simulink model "Symmetry_COPY"  (Simulink 8.1)
settings: Solver=ode23t  StartTime=0.0  StopTime=tfin  RelTol=1e-4
values from neighbouring files (symbols this model uses):
  amp_feedback_saturation = 400    [Symmetry_ini_COPY.m]
  Butterworth_filter_order = 8    [Sketch_controller_model_ini.m]    (also in Symmetry_ini.m; Symmetry_ini_COPY.m)
  C_Network = [0, 0, 0]    [Symmetry_ini.m]    (also in Symmetry_ini_COPY.m)
  Capacitive_Load_R_RC = [30e-3,  60e-3,  40e-3;                                1e-3, 5e-3, 3e-3]    [Symmetry_ini.m]    (also in Symmetry_ini_COPY.m = [60e-3,  120e-3,  80e-3;                                1e-3)
  Capacitive_Load_R_Switching_Sequence = Capacitive_Load_R_Switching_Sequence_'    [Symmetry_ini.m]    (also in Symmetry_ini_COPY.m = ones(3,tfin/Capacitive_Load_R_Switching_Speed(1))')
  Capacitive_Load_R_Switching_Speed = [0.01,0.01,0.01]    [Symmetry_ini.m]    (also in Symmetry_ini_COPY.m)
  Capacitive_Load_S_RC = [30e-3,  60e-3,  40e-3;                                1e-3, 5e-3, 3e-3]    [Symmetry_ini.m]    (also in Symmetry_ini_COPY.m = [60e-3,  120e-3,  80e-3;                                1e-3)
  Capacitive_Load_S_Switching_Sequence = Capacitive_Load_S_Switching_Sequence_'    [Symmetry_ini.m]    (also in Symmetry_ini_COPY.m = ones(3,tfin/Capacitive_Load_R_Switching_Speed(1))')
  Capacitive_Load_S_Switching_Speed = [0.01,0.01,0.01]    [Symmetry_ini.m]    (also in Symmetry_ini_COPY.m)
  Capacitive_Load_T_RC = [30e-3,  60e-3,  40e-3;                                1e-3, 5e-3, 3e-3]    [Symmetry_ini.m]    (also in Symmetry_ini_COPY.m = [60e-3,  120e-3,  80e-3;                                1e-3)
  Capacitive_Load_T_Switching_Sequence = Capacitive_Load_T_Switching_Sequence_'    [Symmetry_ini.m]    (also in Symmetry_ini_COPY.m = ones(3,tfin/Capacitive_Load_R_Switching_Speed(1))')
  Capacitive_Load_T_Switching_Speed = [0.01,0.01,0.01]    [Symmetry_ini.m]    (also in Symmetry_ini_COPY.m)
  i = str2num(answer{1})/sample    [Test_intersect.m]
  initial_value = [1,1,1,                  0,-2/3*pi,-4/3*pi]    [Symmetry_ini_COPY.m]
  L_Network = [3.185e-3, 3.185e-3, 3.185e-3, 3.185e-3]    [Symmetry_ini.m]    (also in Symmetry_ini_COPY.m)
  L_Source = [3.185e-3, 3.185e-3, 3.185e-3]    [Sketch_controller_model_ini.m]    (also in Symmetry_ini.m; Symmetry_ini_COPY.m)
  Load_R = [50,50,50]    [Symmetry_ini.m]    (also in Symmetry_ini_COPY.m)
  Load_RL = [35.35,   35.35,   35.35;                  0.1125,  0.1125,  0.1125]    [Symmetry_ini.m]    (also in Symmetry_ini_COPY.m)
  Load_Wire_Resistance = [0.1,0.2]    [Symmetry_ini.m]    (also in Symmetry_ini_COPY.m)
  P_gain = 0.01    [Symmetry_ini_COPY.m]
  phase_feedback_saturation = pi    (= 3.14159265359)    [Symmetry_ini_COPY.m]
  Phase_Source = [0,2/3*pi,4/3*pi]    [Sketch_controller_model_ini.m]    (also in Symmetry_REAL_TIME_ini.m = [0,-2/3*pi,-4/3*pi]; Symmetry_ini.m; Symmetry_ini_COPY.m = [0,-2/3*pi,-4/3*pi])
  R_Network = [0.4, 0.4, 0.4, 0.4]    [Symmetry_ini.m]    (also in Symmetry_ini_COPY.m)
  R_Source = [0.4, 0.4, 0.4]    [Sketch_controller_model_ini.m]    (also in Symmetry_ini.m; Symmetry_ini_COPY.m)
  sample = 10e-5    (= 0.0001)    [Inverter_ini.m]    (also in Sketch_controller_model_ini.m; Symmetry_REAL_TIME_ini.m; Symmetry_ini.m; Symmetry_ini_COPY.m)
  Source_Frequency = [50,50,50]    [Sketch_controller_model_ini.m]    (also in Symmetry_ini.m; Symmetry_ini_COPY.m)
  Start_Control = 0.1    [Symmetry_ini_COPY.m]
  step_size = [5,5,5,                  0.32,0.32,0.32]    [Symmetry_ini_COPY.m]
  Switch_Load_R = [1,1,1]    [Symmetry_ini.m]    (also in Symmetry_ini_COPY.m = [1,0,0])
  Switch_Load_RC = [1,1,1]    [Symmetry_ini.m]    (also in Symmetry_ini_COPY.m = [0,0,1])
  Switch_Load_RL = [1,1,1]    [Symmetry_ini.m]    (also in Symmetry_ini_COPY.m = [0,1,0])
  test_step = [1,1,1,                  0.08,0.08,0.08]    [Symmetry_ini_COPY.m]
  Urms_Source = [230,230,230]    [Sketch_controller_model_ini.m]    (also in Symmetry_REAL_TIME_ini.m; Symmetry_ini.m; Symmetry_ini_COPY.m)
libraries: powerlib x87, simulink x27, powerlib_extras x12, dspsigops x10, commsequence2 x6, dspxfrm3 x3, dsparch4 x3
(part 1 of 2)
settings Model: Creator=gorbep  LastModifiedBy=Neukirchner László
settings SolverCC: ZeroCrossControl=EnableAll  ZeroCrossAlgorithm=Adaptive  SolverResetMethod=Robust
settings DataIOCC: SignalLoggingSaveFormat=Dataset
settings OptimizationCC: ExpressionDepthLimit=128
settings DebuggingCC: UnderspecifiedInitializationDetection=Simplified  FcnCallInpInsideContextMsg=EnableAllAsError  StateNameClashWarn=none
settings GRTTargetCC: CodeReplacementLibrary=None  CombineOutputUpdateFcns=on  CPPClassGenCompliant=on  GRTInterface=off

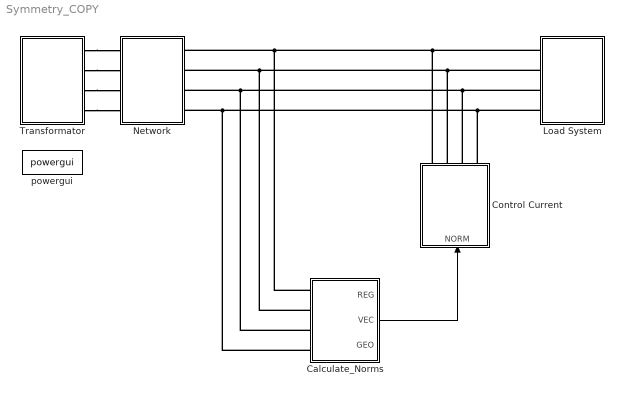
== system Symmetry_COPY ==
  Calculate_Norms : Subsystem
  Control Current : Subsystem
  Load System : Subsystem
  Network : Subsystem
  Transformator : Subsystem
  powergui : powerlib/powergui  SimulationMode=Continuous  SolverType=Tustin  SampleTime=50e-6  frequency=60  SPID=off  DisableSnubberDevices=off  DisableRonSwitches=off  DisableVfSwitches=off  SwTol=0  Interpol=off  DisplayEquations=off  frequencyindice=0  Pbase=100e6  ErrMax=1e-4  Iterations=50  UnitsV=kV  UnitsW=MW  FunctionMessages=off  echomessages=off  HookPort=off  EnableUseOfTLC=off  x0status=blocks  RestoreLinks=warning  ResistiveCurrentMeasurement=off  Frange=[0:2:500]  Ylog=off  Xlog=on  ShowGrid=off  save=off  variable=ZData  structure=0  ZoomFFT=on  StartTime=0.0  cycles=1  DisplayStyle=1  fundamental=60  FreqAxis=off  MaxFrequency=1000  frequencyindicesteady=1  RmsSteady=1  display=off  Ts=0  methode=off
  wires:
  Calculate_Norms/2(VEC) -> Control Current/1(NORM)
  connections:
  Transformator/RConn1 -- Network/LConn1
  Transformator/RConn2 -- Network/LConn2
  Transformator/RConn3 -- Network/LConn3
  Transformator/RConn4 -- Network/LConn4
  Load System/LConn1 -- Calculate_Norms/LConn1 -- Network/RConn1 -- Control Current/RConn1
  Load System/LConn2 -- Calculate_Norms/LConn2 -- Network/RConn2 -- Control Current/RConn2
  Load System/LConn3 -- Calculate_Norms/LConn3 -- Network/RConn3 -- Control Current/RConn3
  Load System/LConn4 -- Network/RConn4 -- Calculate_Norms/LConn4 -- Control Current/RConn4

== system Symmetry_COPY/Calculate_Norms ==
  Gain : Gain  Gain=1e-3
  Gain1 : Gain  Gain=1e-3
  Mearusement_calc : Subsystem
  Sources1 : ToWorkspace  VariableName=V_conn  SampleTime=sample  SaveFormat=Structure With Time
  Sources2 : ToWorkspace  VariableName=angle  SampleTime=sample  SaveFormat=Structure With Time
  Sources3 : ToWorkspace  VariableName=amplitude  SampleTime=sample  SaveFormat=Structure With Time
  Sources4 : ToWorkspace  VariableName=REG  SampleTime=sample  SaveFormat=Structure With Time
  Sources5 : ToWorkspace  VariableName=VEC  SampleTime=sample  SaveFormat=Structure With Time
  Sources6 : ToWorkspace  VariableName=GEO  SampleTime=sample  SaveFormat=Structure With Time
  Voltage Measurement : powerlib/Measurements/Voltage Measurement  PhasorSimulation=off  OutputType=Complex  PSBequivalent=0
  Voltage Measurement1 : powerlib/Measurements/Voltage Measurement  PhasorSimulation=off  OutputType=Complex  PSBequivalent=0
  Voltage Measurement2 : powerlib/Measurements/Voltage Measurement  PhasorSimulation=off  OutputType=Complex  PSBequivalent=0
  R : PMIOPort  Port=1  Side=Left
  S : PMIOPort  Port=2  Side=Left
  T : PMIOPort  Port=3  Side=Left
  N : PMIOPort  Port=4  Side=Left
  REG : Outport
  VEC : Outport  Port=2
  GEO : Outport  Port=3
  wires:
  Voltage Measurement/1 -> Mearusement_calc/1(V_R)
  Voltage Measurement1/1 -> Mearusement_calc/2(V_S)
  Voltage Measurement2/1 -> Mearusement_calc/3(V_T)
  Mearusement_calc/1(Voltage) -> Sources1/1
  Mearusement_calc/2(Amplitude) -> Sources3/1
  Mearusement_calc/3(Angle) -> Sources2/1
  Mearusement_calc/4(Regular) -> REG/1, Sources4/1
  Mearusement_calc/6(Geometrial) -> Gain1/1, Sources6/1
  Mearusement_calc/5(Vectorial) -> Gain/1, Sources5/1
  Gain/1 -> VEC/1
  Gain1/1 -> GEO/1
  connections:
  Voltage Measurement2/LConn1 -- T/RConn1
  Voltage Measurement2/LConn2 -- Voltage Measurement/LConn2 -- Voltage Measurement1/LConn2 -- N/RConn1
  Voltage Measurement/LConn1 -- R/RConn1
  Voltage Measurement1/LConn1 -- S/RConn1

== system Symmetry_COPY/Control Current ==
  NORM : Inport
  Current_Sources : Subsystem
  MATLAB Function : MATLAB Function  TreatAsAtomicUnit=on
  Mux2 : Mux  Inputs=3
  Mux4 : Mux  Inputs=3
  Subsystem : Subsystem
  t : Clock
      settings: Decimation=CLK
  U : PMIOPort  Port=1  Side=Right
  V : PMIOPort  Port=2  Side=Right
  W : PMIOPort  Port=3  Side=Right
  n : PMIOPort  Port=4  Side=Right
  wires:
  t/1 -> MATLAB Function/3(t)
  MATLAB Function/1(CC) -> Current_Sources/1(In1)
  NORM/1 -> Subsystem/1(Norm)
  Subsystem/1(CC_amp_R) -> Mux2/1
  Subsystem/2(CC_amp_S) -> Mux2/2
  Subsystem/3(CC_amp_T) -> Mux2/3
  Subsystem/4(CC_phase_R) -> Mux4/1
  Subsystem/5(CC_phase_R1) -> Mux4/2
  Subsystem/6(CC_phase_R2) -> Mux4/3
  Mux2/1 -> MATLAB Function/1(amp)
  Mux4/1 -> MATLAB Function/2(phase)
  connections:
  U/RConn1 -- Current_Sources/RConn1
  V/RConn1 -- Current_Sources/RConn2
  W/RConn1 -- Current_Sources/RConn3
  n/RConn1 -- Current_Sources/RConn4

== system Symmetry_COPY/Load System ==
  Conncection_Measurements : Subsystem
  Loads : Subsystem
  Log_Signals : Subsystem
  Wire_resistance_1 : Subsystem
  Wire_resistance_2 : Subsystem
  R : PMIOPort  Port=1  Side=Left
  S : PMIOPort  Port=2  Side=Left
  T : PMIOPort  Port=3  Side=Left
  N : PMIOPort  Port=4  Side=Left
  wires:
  Conncection_Measurements/2(I_abc) -> Log_Signals/2(I_ABC)
  Conncection_Measurements/1(V_abc) -> Log_Signals/1(V_ABC)
  Conncection_Measurements/3(V_line-to-line) -> Log_Signals/3(V_line-to-line)
  connections:
  Conncection_Measurements/RConn1 -- Wire_resistance_2/LConn1
  Conncection_Measurements/RConn2 -- Wire_resistance_2/LConn2
  Conncection_Measurements/RConn3 -- Wire_resistance_2/LConn3
  Wire_resistance_1/LConn1 -- R/RConn1
  Wire_resistance_1/LConn2 -- S/RConn1
  Wire_resistance_1/LConn3 -- T/RConn1
  Wire_resistance_1/LConn4 -- N/RConn1
  Conncection_Measurements/LConn1 -- Wire_resistance_1/RConn1
  Conncection_Measurements/LConn2 -- Wire_resistance_1/RConn2
  Conncection_Measurements/LConn3 -- Wire_resistance_1/RConn3
  Wire_resistance_2/RConn1 -- Loads/LConn1
  Wire_resistance_2/RConn2 -- Loads/LConn2
  Wire_resistance_2/RConn3 -- Loads/LConn3
  Wire_resistance_2/RConn4 -- Loads/LConn4
  Wire_resistance_1/RConn4 -- Conncection_Measurements/LConn4
  Wire_resistance_2/LConn4 -- Conncection_Measurements/RConn4

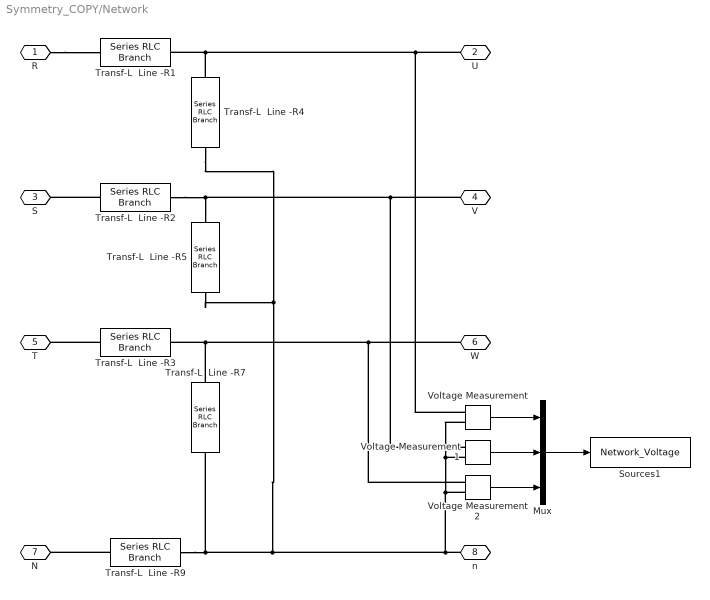
== system Symmetry_COPY/Network ==
  Mux : Mux  Inputs=3
  Sources1 : ToWorkspace  VariableName=Network_Voltage  SampleTime=-1  SaveFormat=Structure With Time
  Transf-L  Line -R1 : powerlib/Elements/Series RLC Branch  LConnTagsString=__new0  RConnTagsString=__new0  BranchType=RL  Resistance=R_Network(1)  Inductance=L_Network(1)  SetiL0=off  InitialCurrent=0  Capacitance=1.0  Setx0=off  InitialVoltage=0  Measurements=None
  Transf-L  Line -R2 : powerlib/Elements/Series RLC Branch  LConnTagsString=__new0  RConnTagsString=__new0  BranchType=RL  Resistance=R_Network(2)  Inductance=L_Network(2)  SetiL0=off  InitialCurrent=0  Capacitance=1.0  Setx0=off  InitialVoltage=0  Measurements=None
  Transf-L  Line -R3 : powerlib/Elements/Series RLC Branch  LConnTagsString=__new0  RConnTagsString=__new0  BranchType=RL  Resistance=R_Network(3)  Inductance=L_Network(3)  SetiL0=off  InitialCurrent=0  Capacitance=1.0  Setx0=off  InitialVoltage=0  Measurements=None
  Transf-L  Line -R4 : powerlib/Elements/Series RLC Branch  LConnTagsString=__new0  RConnTagsString=__new0  BranchType=C  Resistance=i  Inductance=0.003185  SetiL0=off  InitialCurrent=0  Capacitance=C_Network(1)  Setx0=off  InitialVoltage=0  Measurements=None
  Transf-L  Line -R5 : powerlib/Elements/Series RLC Branch  LConnTagsString=__new0  RConnTagsString=__new0  BranchType=C  Resistance=i  Inductance=0.003185  SetiL0=off  InitialCurrent=0  Capacitance=C_Network(2)  Setx0=off  InitialVoltage=0  Measurements=None
  Transf-L  Line -R7 : powerlib/Elements/Series RLC Branch  LConnTagsString=__new0  RConnTagsString=__new0  BranchType=C  Resistance=i  Inductance=0.003185  SetiL0=off  InitialCurrent=0  Capacitance=C_Network(2)  Setx0=off  InitialVoltage=0  Measurements=None
  Transf-L  Line -R9 : powerlib/Elements/Series RLC Branch  LConnTagsString=__new0  RConnTagsString=__new0  BranchType=RL  Resistance=R_Network(4)  Inductance=L_Network(4)  SetiL0=off  InitialCurrent=0  Capacitance=1.0  Setx0=off  InitialVoltage=0  Measurements=None
  Voltage Measurement : powerlib/Measurements/Voltage Measurement  PhasorSimulation=off  OutputType=Complex  PSBequivalent=0
  Voltage Measurement1 : powerlib/Measurements/Voltage Measurement  PhasorSimulation=off  OutputType=Complex  PSBequivalent=0
  Voltage Measurement2 : powerlib/Measurements/Voltage Measurement  PhasorSimulation=off  OutputType=Complex  PSBequivalent=0
  R : PMIOPort  Port=1  Side=Left
  U : PMIOPort  Port=2  Side=Right
  S : PMIOPort  Port=3  Side=Left
  V : PMIOPort  Port=4  Side=Right
  T : PMIOPort  Port=5  Side=Left
  W : PMIOPort  Port=6  Side=Right
  N : PMIOPort  Port=7  Side=Left
  n : PMIOPort  Port=8  Side=Right
  wires:
  Voltage Measurement/1 -> Mux/1
  Voltage Measurement1/1 -> Mux/2
  Voltage Measurement2/1 -> Mux/3
  Mux/1 -> Sources1/1
  connections:
  Transf-L  Line -R4/LConn1 -- Voltage Measurement/LConn1 -- U/RConn1 -- Transf-L  Line -R1/RConn1
  Transf-L  Line -R2/RConn1 -- Voltage Measurement1/LConn1 -- V/RConn1 -- Transf-L  Line -R5/LConn1
  Transf-L  Line -R7/LConn1 -- Voltage Measurement2/LConn1 -- W/RConn1 -- Transf-L  Line -R3/RConn1
  Transf-L  Line -R3/LConn1 -- T/RConn1
  Transf-L  Line -R2/LConn1 -- S/RConn1
  R/RConn1 -- Transf-L  Line -R1/LConn1
  Voltage Measurement/LConn2 -- Voltage Measurement1/LConn2 -- Transf-L  Line -R7/RConn1 -- Transf-L  Line -R9/RConn1 -- Transf-L  Line -R4/RConn1 -- Transf-L  Line -R5/RConn1 -- n/RConn1 -- Voltage Measurement2/LConn2
  Transf-L  Line -R9/LConn1 -- N/RConn1

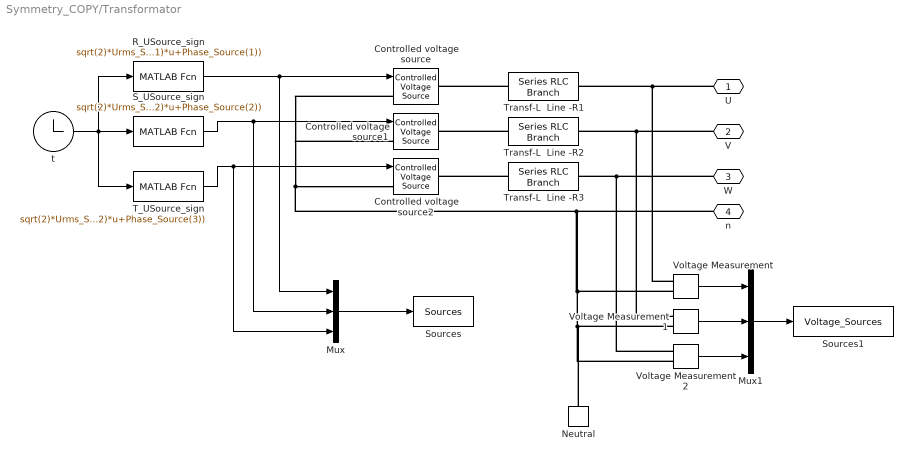
== system Symmetry_COPY/Transformator ==
  " R_USource_sign" : MATLABFcn  MATLABFcn=sqrt(2)*Urms_Source(1)*sin(2*pi*Source_Frequency(1)*u+Phase_Source(1))  SampleTime=sample
  " S_USource_sign" : MATLABFcn  MATLABFcn=sqrt(2)*Urms_Source(2)*sin(2*pi*Source_Frequency(2)*u+Phase_Source(2))  SampleTime=sample
  " T_USource_sign" : MATLABFcn  MATLABFcn=sqrt(2)*Urms_Source(3)*sin(2*pi*Source_Frequency(2)*u+Phase_Source(3))  SampleTime=sample
  Controlled voltage source : powerlib/Electrical Sources/Controlled Voltage Source  Initialize=off  Source_Type=AC  Amplitude=0  Phase=0  Frequency=0  Measurements=None
  Controlled voltage source1 : powerlib/Electrical Sources/Controlled Voltage Source  Initialize=off  Source_Type=AC  Amplitude=0  Phase=0  Frequency=0  Measurements=None
  Controlled voltage source2 : powerlib/Electrical Sources/Controlled Voltage Source  Initialize=off  Source_Type=AC  Amplitude=0  Phase=0  Frequency=0  Measurements=None
  Mux : Mux  Inputs=3
  Mux1 : Mux  Inputs=3
  Neutral : powerlib/Elements/Neutral  LConnTagsString=a  NodeNumber=10
  Sources : ToWorkspace  VariableName=Sources  SampleTime=-1  SaveFormat=Structure With Time
  Sources1 : ToWorkspace  VariableName=Voltage_Sources  SampleTime=-1  SaveFormat=Structure With Time
  Transf-L  Line -R1 : powerlib/Elements/Series RLC Branch  LConnTagsString=__new0  RConnTagsString=__new0  BranchType=RL  Resistance=R_Source(1)  Inductance=L_Source(1)  SetiL0=off  InitialCurrent=0  Capacitance=1.0  Setx0=off  InitialVoltage=0  Measurements=None
  Transf-L  Line -R2 : powerlib/Elements/Series RLC Branch  LConnTagsString=__new0  RConnTagsString=__new0  BranchType=RL  Resistance=R_Source(2)  Inductance=L_Source(2)  SetiL0=off  InitialCurrent=0  Capacitance=1.0  Setx0=off  InitialVoltage=0  Measurements=None
  Transf-L  Line -R3 : powerlib/Elements/Series RLC Branch  LConnTagsString=__new0  RConnTagsString=__new0  BranchType=RL  Resistance=R_Source(3)  Inductance=L_Source(3)  SetiL0=off  InitialCurrent=0  Capacitance=1.0  Setx0=off  InitialVoltage=0  Measurements=None
  Voltage Measurement : powerlib/Measurements/Voltage Measurement  PhasorSimulation=off  OutputType=Complex  PSBequivalent=0
  Voltage Measurement1 : powerlib/Measurements/Voltage Measurement  PhasorSimulation=off  OutputType=Complex  PSBequivalent=0
  Voltage Measurement2 : powerlib/Measurements/Voltage Measurement  PhasorSimulation=off  OutputType=Complex  PSBequivalent=0
  t : Clock
      settings: Decimation=CLK
  U : PMIOPort  Port=1  Side=Right
  V : PMIOPort  Port=2  Side=Right
  W : PMIOPort  Port=3  Side=Right
  n : PMIOPort  Port=4  Side=Right
  wires:
  Mux/1 -> Sources/1
  " R_USource_sign"/1 -> Mux/1, Controlled voltage source/1
  " S_USource_sign"/1 -> Mux/2, Controlled voltage source1/1
  " T_USource_sign"/1 -> Mux/3, Controlled voltage source2/1
  t/1 -> " R_USource_sign"/1, " T_USource_sign"/1, " S_USource_sign"/1
  Voltage Measurement/1 -> Mux1/1
  Voltage Measurement1/1 -> Mux1/2
  Voltage Measurement2/1 -> Mux1/3
  Mux1/1 -> Sources1/1
  connections:
  n/RConn1 -- Neutral/LConn1 -- Voltage Measurement2/LConn2 -- Voltage Measurement1/LConn2 -- Voltage Measurement/LConn2 -- Controlled voltage source/LConn1 -- Controlled voltage source1/LConn1 -- Controlled voltage source2/LConn1
  Transf-L  Line -R2/LConn1 -- Controlled voltage source1/RConn1
  Transf-L  Line -R3/LConn1 -- Controlled voltage source2/RConn1
  Transf-L  Line -R1/LConn1 -- Controlled voltage source/RConn1
  U/RConn1 -- Voltage Measurement/LConn1 -- Transf-L  Line -R1/RConn1
  V/RConn1 -- Voltage Measurement1/LConn1 -- Transf-L  Line -R2/RConn1
  W/RConn1 -- Voltage Measurement2/LConn1 -- Transf-L  Line -R3/RConn1

== system Symmetry_COPY/Calculate_Norms/Mearusement_calc ==
  V_R : Inport
  V_S : Inport  Port=2
  V_T : Inport  Port=3
  Demux{1..6} (6 alike) : Demux  Outputs=3
  FFT : Subsystem
  Mux1 : Mux  Inputs=3
  geometrial norm1 : MATLAB Function  TreatAsAtomicUnit=on
  regular norm : MATLAB Function  TreatAsAtomicUnit=on
  vectorial norm : MATLAB Function  TreatAsAtomicUnit=on
  Voltage : Outport
  Amplitude : Outport  Port=2
  Angle : Outport  Port=3
  Regular : Outport  Port=4
  Vectorial : Outport  Port=5
  Geometrial : Outport  Port=6
  wires:
  V_R/1 -> Mux1/1
  V_T/1 -> Mux1/3
  Mux1/1 -> Voltage/1, FFT/1(Voltage_3Phase)
  V_S/1 -> Mux1/2
  regular norm/1(REG_norm) -> Regular/1
  Demux2/1 -> regular norm/1(amplitude_R)
  Demux2/2 -> regular norm/2(amplitude_S)
  Demux2/3 -> regular norm/3(amplitude_T)
  Demux3/1 -> regular norm/4(phase_R)
  Demux3/2 -> regular norm/5(phase_S)
  Demux3/3 -> regular norm/6(phase_T)
  Demux1/1 -> vectorial norm/1(amplitude_R)
  Demux1/2 -> vectorial norm/2(amplitude_S)
  Demux1/3 -> vectorial norm/3(amplitude_T)
  Demux4/1 -> vectorial norm/4(phase_R)
  Demux4/2 -> vectorial norm/5(phase_S)
  Demux4/3 -> vectorial norm/6(phase_T)
  vectorial norm/1(VEC_norm) -> Vectorial/1
  FFT/1(Amplitude) -> Amplitude/1, Demux5/1, Demux1/1, Demux2/1
  FFT/2(Phase_in_rad) -> Angle/1, Demux6/1, Demux4/1, Demux3/1
  Demux5/1 -> geometrial norm1/1(amplitude_R)
  Demux5/2 -> geometrial norm1/2(amplitude_S)
  Demux5/3 -> geometrial norm1/3(amplitude_T)
  Demux6/1 -> geometrial norm1/4(phase_R)
  Demux6/2 -> geometrial norm1/5(phase_S)
  Demux6/3 -> geometrial norm1/6(phase_T)
  geometrial norm1/1(GEO_norm) -> Geometrial/1

== system Symmetry_COPY/Control Current/Current_Sources ==
  In1 : Inport
  Controlled Current Source : powerlib/Electrical Sources/Controlled Current Source  Initialize=on  Source_Type=AC  Amplitude=0  Phase=0  Frequency=0  Measurements=None
  Controlled Current Source1 : powerlib/Electrical Sources/Controlled Current Source  Initialize=on  Source_Type=AC  Amplitude=0  Phase=0  Frequency=0  Measurements=None
  Controlled Current Source2 : powerlib/Electrical Sources/Controlled Current Source  Initialize=on  Source_Type=AC  Amplitude=0  Phase=0  Frequency=0  Measurements=None
  Demux : Demux  Outputs=3
  M3 : powerlib/Measurements/Three-Phase V-I Measurement  VoltageMeasurement=no  SetLabelV=off  LabelV=V_RST  Vpu=off  VpuLL=off  CurrentMeasurement=yes  SetLabelI=off  LabelI=I_RST  Ipu=off  Pbase=100e6  Vbase=500e3  OutputType=Complex  PhasorSimulation=off  PSBequivalent=0
  P(t) Filter : dsparch4/Analog Filter Design  method=Butterworth  filttype=Lowpass  N=Butterworth_filter_order  Wlo=Butterworth_passband_frequency  Whi=80  Rp=2  Rs=40
  P(t) Filter1 : dsparch4/Analog Filter Design  method=Butterworth  filttype=Lowpass  N=Butterworth_filter_order  Wlo=Butterworth_passband_frequency  Whi=80  Rp=2  Rs=40
  P(t) Filter2 : dsparch4/Analog Filter Design  method=Butterworth  filttype=Lowpass  N=Butterworth_filter_order  Wlo=Butterworth_passband_frequency  Whi=80  Rp=2  Rs=40
  Sources1 : ToWorkspace  VariableName=CC  SampleTime=sample  SaveFormat=Structure With Time
  Conn1 : PMIOPort  Port=1  Side=Right
  Conn2 : PMIOPort  Port=2  Side=Right
  Conn3 : PMIOPort  Port=3  Side=Right
  Conn4 : PMIOPort  Port=4  Side=Right
  wires:
  M3/1 -> Sources1/1
  In1/1 -> Demux/1
  Demux/1 -> P(t) Filter/1
  Demux/2 -> P(t) Filter1/1
  Demux/3 -> P(t) Filter2/1
  P(t) Filter/1 -> Controlled Current Source/1
  P(t) Filter1/1 -> Controlled Current Source1/1
  P(t) Filter2/1 -> Controlled Current Source2/1
  connections:
  Controlled Current Source/LConn1 -- Controlled Current Source1/LConn1 -- Conn4/RConn1 -- Controlled Current Source2/LConn1
  M3/LConn1 -- Controlled Current Source/RConn1
  M3/LConn2 -- Controlled Current Source1/RConn1
  M3/LConn3 -- Controlled Current Source2/RConn1
  Conn1/RConn1 -- M3/RConn1
  Conn2/RConn1 -- M3/RConn2
  Conn3/RConn1 -- M3/RConn3

== system Symmetry_COPY/Control Current/Subsystem ==
  Norm : Inport
  Create_Date : Subsystem
  Mux : Mux  Inputs=3
  Mux1 : Mux  Inputs=3
  Phase_control_S : Subsystem
  Scope : Scope
      settings: SaveName=ScopeData2
  Scope1 : Scope
      settings: SaveName=ScopeData3
  amp_control_R : Subsystem
  amp_control_S : Subsystem
  amp_control_T : Subsystem
  phase_control_R : Subsystem
  phase_control_T : Subsystem
  CC_amp_R : Outport
  CC_amp_S : Outport  Port=2
  CC_amp_T : Outport  Port=3
  CC_phase_R : Outport  Port=4
  CC_phase_R1 : Outport  Port=5
  CC_phase_R2 : Outport  Port=6
  wires:
  amp_control_S/1(amp_S) -> Mux/2, CC_amp_S/1
  amp_control_T/1(amp_T) -> Mux/3, CC_amp_T/1
  Create_Date/1(Controller_data) -> phase_control_T/1(Control), Phase_control_S/1(Control), phase_control_R/1(Control), amp_control_T/1(Control), amp_control_S/1(Control), amp_control_R/1(Control)
  Norm/1 -> Create_Date/1(NORM)
  Mux/1 -> Scope/1
  amp_control_R/1(amp_R) -> Mux/1, CC_amp_R/1
  Phase_control_S/1(phase_S) -> Mux1/2, CC_phase_R1/1
  phase_control_T/1(phase_S) -> Mux1/3, CC_phase_R2/1
  Mux1/1 -> Scope1/1
  phase_control_R/1(phase_R) -> Mux1/1, CC_phase_R/1

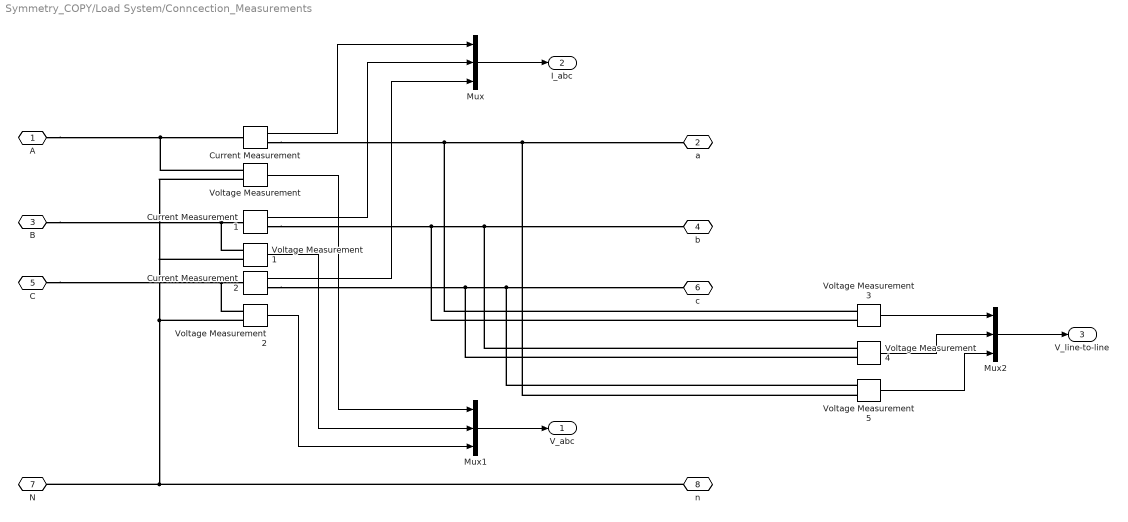
== system Symmetry_COPY/Load System/Conncection_Measurements ==
  Current Measurement : powerlib/Measurements/Current Measurement  PhasorSimulation=off  OutputType=Complex  PSBequivalent=0
  Current Measurement1 : powerlib/Measurements/Current Measurement  PhasorSimulation=off  OutputType=Complex  PSBequivalent=0
  Current Measurement2 : powerlib/Measurements/Current Measurement  PhasorSimulation=off  OutputType=Complex  PSBequivalent=0
  Mux : Mux  Inputs=3
  Mux1 : Mux  Inputs=3
  Mux2 : Mux  Inputs=3
  Voltage Measurement{,1..5} (6 alike) : powerlib/Measurements/Voltage Measurement  PhasorSimulation=off  OutputType=Complex  PSBequivalent=0
  A : PMIOPort  Port=1  Side=Left
  a : PMIOPort  Port=2  Side=Right
  B : PMIOPort  Port=3  Side=Left
  b : PMIOPort  Port=4  Side=Right
  C : PMIOPort  Port=5  Side=Left
  c : PMIOPort  Port=6  Side=Right
  N : PMIOPort  Port=7  Side=Left
  n : PMIOPort  Port=8  Side=Right
  V_abc : Outport
  I_abc : Outport  Port=2
  V_line-to-line : Outport  Port=3
  wires:
  Current Measurement1/1 -> Mux/2
  Mux1/1 -> V_abc/1
  Mux/1 -> I_abc/1
  Current Measurement/1 -> Mux/1
  Voltage Measurement/1 -> Mux1/1
  Current Measurement2/1 -> Mux/3
  Voltage Measurement1/1 -> Mux1/2
  Voltage Measurement2/1 -> Mux1/3
  Mux2/1 -> V_line-to-line/1
  Voltage Measurement3/1 -> Mux2/1
  Voltage Measurement4/1 -> Mux2/2
  Voltage Measurement5/1 -> Mux2/3
  connections:
  Current Measurement2/RConn1 -- Voltage Measurement4/LConn2 -- Voltage Measurement5/LConn1 -- c/RConn1
  Current Measurement/RConn1 -- Voltage Measurement5/LConn2 -- a/RConn1 -- Voltage Measurement3/LConn1
  Current Measurement1/RConn1 -- Voltage Measurement4/LConn1 -- b/RConn1 -- Voltage Measurement3/LConn2
  Voltage Measurement2/LConn1 -- Current Measurement2/LConn1 -- C/RConn1
  Voltage Measurement2/LConn2 -- N/RConn1 -- n/RConn1 -- Voltage Measurement1/LConn2 -- Voltage Measurement/LConn2
  Voltage Measurement1/LConn1 -- Current Measurement1/LConn1 -- B/RConn1
  Voltage Measurement/LConn1 -- A/RConn1 -- Current Measurement/LConn1

== system Symmetry_COPY/Load System/Loads ==
  Capacitive_Loads_RST : Subsystem
  Inductive_Loads_RST : Subsystem
  Ohmic_Loads_RST : Subsystem
  R : PMIOPort  Port=1  Side=Left
  S : PMIOPort  Port=2  Side=Left
  T : PMIOPort  Port=3  Side=Left
  N : PMIOPort  Port=4  Side=Left
  connections:
  Ohmic_Loads_RST/LConn1 -- R/RConn1 -- Inductive_Loads_RST/LConn1 -- Capacitive_Loads_RST/RConn1
  Capacitive_Loads_RST/RConn2 -- S/RConn1 -- Inductive_Loads_RST/LConn2 -- Ohmic_Loads_RST/LConn2
  Capacitive_Loads_RST/RConn3 -- T/RConn1 -- Inductive_Loads_RST/LConn3 -- Ohmic_Loads_RST/LConn3
  N/RConn1 -- Inductive_Loads_RST/RConn1 -- Ohmic_Loads_RST/RConn1 -- Capacitive_Loads_RST/LConn1

== system Symmetry_COPY/Load System/Log_Signals ==
  V_ABC : Inport
  I_ABC : Inport  Port=2
  V_line-to-line : Inport  Port=3
  3_Phase_P_Q : Subsystem
  3_Phase_RMS : Subsystem
  3_Phase_RMS1 : Subsystem
  3_Phase_THD : Subsystem
  Sources1 : ToWorkspace  VariableName=V  SampleTime=sample  SaveFormat=Structure With Time
  Sources2 : ToWorkspace  VariableName=Vrms  SampleTime=sample  SaveFormat=Structure With Time
  Sources3 : ToWorkspace  VariableName=V_line  SampleTime=sample  SaveFormat=Structure With Time
  To Workspace : ToWorkspace  VariableName=Connection_Current_RST  SampleTime=sample  SaveFormat=Timeseries
  To Workspace1 : ToWorkspace  VariableName=Connection_Currnet_RMS_RST  SampleTime=sample  SaveFormat=Timeseries
  To Workspace2 : ToWorkspace  VariableName=Connection_Voltage_THD_RST  SampleTime=sample  SaveFormat=Timeseries
  To Workspace4 : ToWorkspace  VariableName=Connection_Voltage_RMS_RST  SampleTime=sample  SaveFormat=Timeseries
  To Workspace5 : ToWorkspace  VariableName=Connection_Voltage_RST  SampleTime=sample  SaveFormat=Timeseries
  To Workspace6 : ToWorkspace  VariableName=Connection_P_Q_RST  SampleTime=sample  SaveFormat=Timeseries
  wires:
  I_ABC/1 -> 3_Phase_RMS1/1(I_RST), To Workspace/1, 3_Phase_P_Q/2(I_RMS)
  V_ABC/1 -> 3_Phase_RMS/1(U_RST), 3_Phase_THD/1(U_RST), Sources1/1, To Workspace5/1, 3_Phase_P_Q/1(U_RMS)
  3_Phase_RMS1/1(I_RMS) -> To Workspace1/1
  3_Phase_RMS/1(U_RMS) -> Sources2/1, To Workspace4/1
  3_Phase_P_Q/1(P_Q_RMS) -> To Workspace6/1
  3_Phase_THD/1(THD_RST) -> To Workspace2/1
  V_line-to-line/1 -> Sources3/1

== system Symmetry_COPY/Load System/Wire_resistance_1 ==
  Series RLC Branch{,5..7} (4 alike) : powerlib/Elements/Series RLC Branch  LConnTagsString=__new0  RConnTagsString=__new0  BranchType=R  Resistance=Load_Wire_Resistance(1)  Inductance=1e-3  SetiL0=off  InitialCurrent=0  Capacitance=1e-6  Setx0=off  InitialVoltage=0  Measurements=None
  A : PMIOPort  Port=1  Side=Left
  a : PMIOPort  Port=2  Side=Right
  B : PMIOPort  Port=3  Side=Left
  b : PMIOPort  Port=4  Side=Right
  C : PMIOPort  Port=5  Side=Left
  c : PMIOPort  Port=6  Side=Right
  N : PMIOPort  Port=7  Side=Left
  n : PMIOPort  Port=8  Side=Right
  connections:
  Series RLC Branch7/RConn1 -- n/RConn1
  Series RLC Branch5/LConn1 -- B/RConn1
  Series RLC Branch6/LConn1 -- C/RConn1
  Series RLC Branch/RConn1 -- a/RConn1
  Series RLC Branch/LConn1 -- A/RConn1
  Series RLC Branch7/LConn1 -- N/RConn1
  Series RLC Branch6/RConn1 -- c/RConn1
  Series RLC Branch5/RConn1 -- b/RConn1

== system Symmetry_COPY/Load System/Wire_resistance_2 ==
  Series RLC Branch{1..4} (4 alike) : powerlib/Elements/Series RLC Branch  LConnTagsString=__new0  RConnTagsString=__new0  BranchType=R  Resistance=Load_Wire_Resistance(2)  Inductance=1e-3  SetiL0=off  InitialCurrent=0  Capacitance=1e-6  Setx0=off  InitialVoltage=0  Measurements=None
  A : PMIOPort  Port=1  Side=Left
  a : PMIOPort  Port=2  Side=Right
  B : PMIOPort  Port=3  Side=Left
  b : PMIOPort  Port=4  Side=Right
  C : PMIOPort  Port=5  Side=Left
  c : PMIOPort  Port=6  Side=Right
  N : PMIOPort  Port=7  Side=Left
  n : PMIOPort  Port=8  Side=Right
  connections:
  Series RLC Branch2/RConn1 -- b/RConn1
  Series RLC Branch1/RConn1 -- a/RConn1
  Series RLC Branch4/RConn1 -- n/RConn1
  Series RLC Branch2/LConn1 -- B/RConn1
  Series RLC Branch3/RConn1 -- c/RConn1
  Series RLC Branch3/LConn1 -- C/RConn1
  Series RLC Branch1/LConn1 -- A/RConn1
  Series RLC Branch4/LConn1 -- N/RConn1

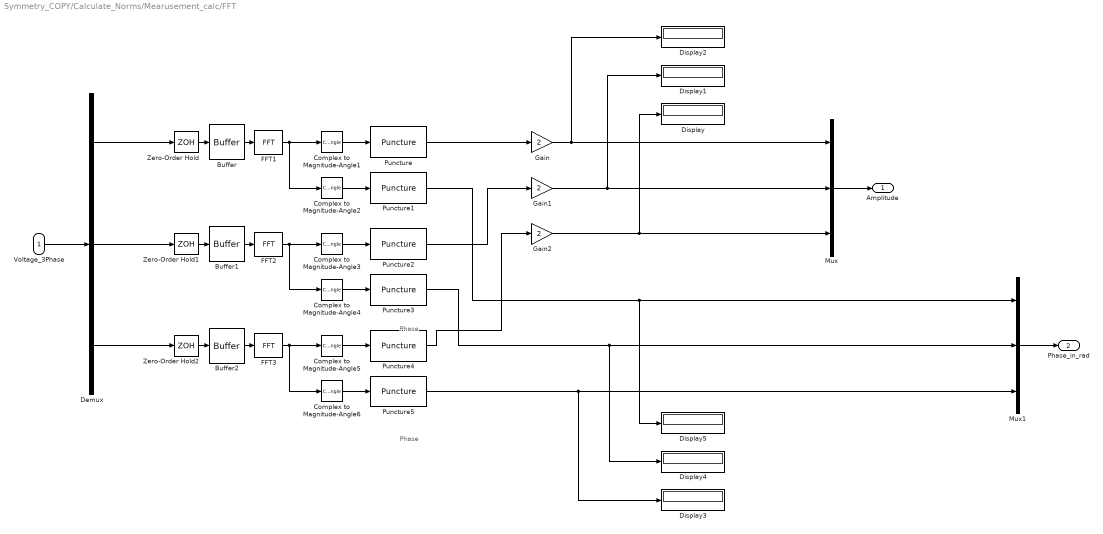
== system Symmetry_COPY/Calculate_Norms/Mearusement_calc/FFT ==
  note: Phase
  note: Phase
  Voltage_3Phase : Inport
  Buffer : Buffer  N=128
  Buffer1 : Buffer  N=128
  Buffer2 : Buffer  N=128
  Complex to Magnitude-Angle1 : ComplexToMagnitudeAngle  Output=Magnitude
  Complex to Magnitude-Angle2 : ComplexToMagnitudeAngle  Output=Angle
  Complex to Magnitude-Angle3 : ComplexToMagnitudeAngle  Output=Magnitude
  Complex to Magnitude-Angle4 : ComplexToMagnitudeAngle  Output=Angle
  Complex to Magnitude-Angle5 : ComplexToMagnitudeAngle  Output=Magnitude
  Complex to Magnitude-Angle6 : ComplexToMagnitudeAngle  Output=Angle
  Demux : Demux  Outputs=3
  Display{,1..5} (6 alike) : Display
  FFT1 : dspxfrm3/FFT  CompMethod=Table lookup  TableOpt=HYBRID  TableOptActive=Speed  BitRevOrder=off  InheritFFTLength=on  FFTLength=64  RowConvenienceOn=on  FFTImplementation=Auto  SkipNorm=on  firstCoeffDataTypeStr=Inherit: Same word length as input  firstCoeffLastDataTypeStr=Inherit: Same word length as input  outputMin=[]  outputMax=[]  roundingMode=Floor  overflowMode=off
  FFT2 : dspxfrm3/FFT  CompMethod=Table lookup  TableOpt=HYBRID  TableOptActive=Speed  BitRevOrder=off  InheritFFTLength=on  FFTLength=64  RowConvenienceOn=on  FFTImplementation=Auto  SkipNorm=on  firstCoeffDataTypeStr=Inherit: Same word length as input  firstCoeffLastDataTypeStr=Inherit: Same word length as input  outputMin=[]  outputMax=[]  roundingMode=Floor  overflowMode=off
  FFT3 : dspxfrm3/FFT  CompMethod=Table lookup  TableOpt=HYBRID  TableOptActive=Speed  BitRevOrder=off  InheritFFTLength=on  FFTLength=64  RowConvenienceOn=on  FFTImplementation=Auto  SkipNorm=on  firstCoeffDataTypeStr=Inherit: Same word length as input  firstCoeffLastDataTypeStr=Inherit: Same word length as input  outputMin=[]  outputMax=[]  roundingMode=Floor  overflowMode=off
  Gain : Gain  Gain=2  SampleTime=sample
  Gain1 : Gain  Gain=2  SampleTime=sample
  Gain2 : Gain  Gain=2  SampleTime=sample
  Mux : Mux  Inputs=3
  Mux1 : Mux  Inputs=3
  Puncture{,1..5} (6 alike) : commsequence2/Puncture  punctureVector=s'
  Zero-Order Hold : ZeroOrderHold  SampleTime=20e-3/128
  Zero-Order Hold1 : ZeroOrderHold  SampleTime=20e-3/128
  Zero-Order Hold2 : ZeroOrderHold  SampleTime=20e-3/128
  Amplitude : Outport
  Phase_in_rad : Outport  Port=2
  wires:
  FFT1/1 -> Complex to Magnitude-Angle1/1, Complex to Magnitude-Angle2/1
  Buffer/1 -> FFT1/1
  Zero-Order Hold/1 -> Buffer/1
  Complex to Magnitude-Angle1/1 -> Puncture/1
  Complex to Magnitude-Angle2/1 -> Puncture1/1
  FFT2/1 -> Complex to Magnitude-Angle4/1, Complex to Magnitude-Angle3/1
  Buffer1/1 -> FFT2/1
  Zero-Order Hold1/1 -> Buffer1/1
  Complex to Magnitude-Angle3/1 -> Puncture2/1
  Complex to Magnitude-Angle4/1 -> Puncture3/1
  FFT3/1 -> Complex to Magnitude-Angle5/1, Complex to Magnitude-Angle6/1
  Buffer2/1 -> FFT3/1
  Zero-Order Hold2/1 -> Buffer2/1
  Complex to Magnitude-Angle5/1 -> Puncture4/1
  Complex to Magnitude-Angle6/1 -> Puncture5/1
  Voltage_3Phase/1 -> Demux/1
  Demux/2 -> Zero-Order Hold1/1
  Demux/3 -> Zero-Order Hold2/1
  Puncture/1 -> Gain/1
  Puncture2/1 -> Gain1/1
  Puncture4/1 -> Gain2/1
  Puncture1/1 -> Display5/1, Mux1/1
  Puncture3/1 -> Display4/1, Mux1/2
  Puncture5/1 -> Display3/1, Mux1/3
  Mux/1 -> Amplitude/1
  Mux1/1 -> Phase_in_rad/1
  Gain/1 -> Display2/1, Mux/1
  Gain1/1 -> Display1/1, Mux/2
  Gain2/1 -> Display/1, Mux/3
  Demux/1 -> Zero-Order Hold/1

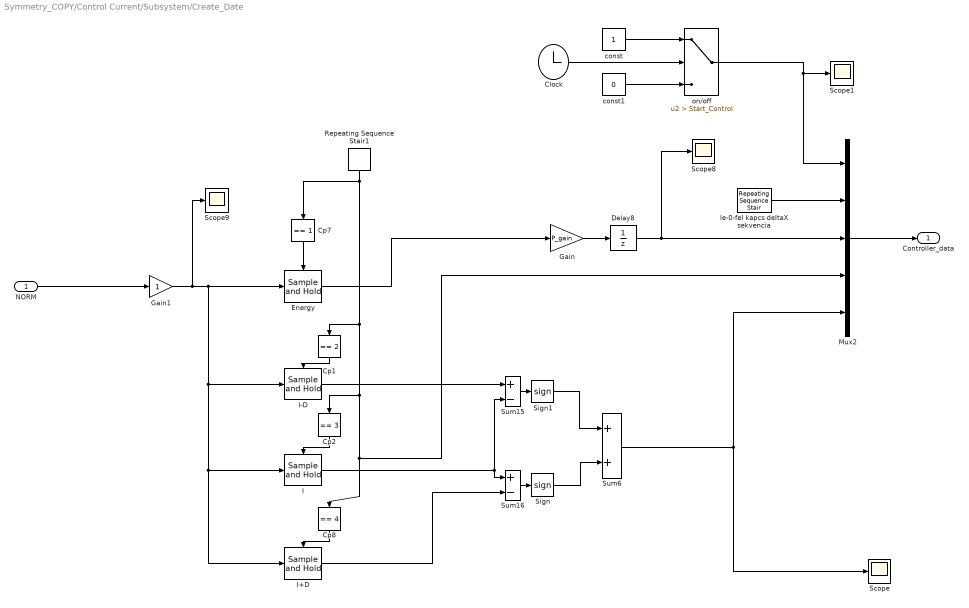
== system Symmetry_COPY/Control Current/Subsystem/Create_Date ==
  NORM : Inport
  Clock : Clock
      settings: Decimation=CLK
  Cp1 : simulink/Logic and Bit Operations/Compare To Constant  relop===  const=2  OutDataTypeStr=uint8  ZeroCross=off
  Cp2 : simulink/Logic and Bit Operations/Compare To Constant  relop===  const=3  OutDataTypeStr=uint8  ZeroCross=off
  Cp7 : simulink/Logic and Bit Operations/Compare To Constant  relop===  const=1  OutDataTypeStr=uint8  ZeroCross=off
  Cp8 : simulink/Logic and Bit Operations/Compare To Constant  relop===  const=4  OutDataTypeStr=uint8  ZeroCross=off
  Delay8 : UnitDelay  SampleTime=sample
  Energy : dspsigops/Sample and Hold  trig=Rising edge  initCond=18  latchinput=off
  Gain : Gain  Gain=P_gain
  Gain1 : Gain
  I : dspsigops/Sample and Hold  trig=Rising edge  initCond=0  latchinput=off
  I+D : dspsigops/Sample and Hold  trig=Rising edge  initCond=0  latchinput=off
  I-D : dspsigops/Sample and Hold  trig=Rising edge  initCond=0  latchinput=off
  Mux2 : Mux  Inputs=5
  Repeating Sequence Stair1 : simulink/Sources/Repeating Sequence Stair  OutValues=[1 2 3 4 5].'  tsamp=0.02  OutMin=[]  OutMax=[]  OutDataTypeStr=float('double')  OutputDataTypeScalingMode=Specify via dialog  OutDataType=float('double')  ConRadixGroup=Best Precision: Vector-wise  OutScaling=2^-12
  Scope{,1,8..9} (4 alike) : Scope
      Scope1 settings: SaveName=ScopeData7
      Scope8 settings: SaveName=ScopeData8
      Scope9 settings: SaveName=ScopeData9
  Sign : Signum
  Sign1 : Signum
  Sum15 : Sum  Inputs=+-
  Sum16 : Sum  Inputs=+-
  Sum6 : Sum
  const : Constant
  const1 : Constant  Value=0
  le-0-fel kapcs deltaX sekvencia : simulink/Sources/Repeating Sequence Stair  OutValues=[-1 0 1 0 0].'  tsamp=0.02  OutMin=[]  OutMax=[]  OutDataTypeStr=float('double')  OutputDataTypeScalingMode=Specify via dialog  OutDataType=float('double')  ConRadixGroup=Best Precision: Vector-wise  OutScaling=2^-12
  on/off : Switch  Criteria=u2 > Threshold  Threshold=Start_Control
  Controller_data : Outport
  wires:
  Cp1/1 -> I-D/Trigger
  Repeating Sequence Stair1/1 -> Cp7/1, Mux2/4, Cp8/1, Cp2/1, Cp1/1
  Cp7/1 -> Energy/Trigger
  Energy/1 -> Gain/1
  Cp2/1 -> I/Trigger
  Cp8/1 -> I+D/Trigger
  Gain1/1 -> Scope9/1, I+D/1, I/1, I-D/1, Energy/1
  I-D/1 -> Sum15/1
  I/1 -> Sum15/2, Sum16/1
  I+D/1 -> Sum16/2
  Sum16/1 -> Sign/1
  Sum15/1 -> Sign1/1
  Gain/1 -> Delay8/1
  Sign/1 -> Sum6/2
  Sign1/1 -> Sum6/1
  le-0-fel kapcs deltaX sekvencia/1 -> Mux2/2
  Delay8/1 -> Scope8/1, Mux2/3
  on/off/1 -> Scope1/1, Mux2/1
  Mux2/1 -> Controller_data/1
  NORM/1 -> Gain1/1
  const/1 -> on/off/1
  const1/1 -> on/off/3
  Clock/1 -> on/off/2
  Sum6/1 -> Mux2/5, Scope/1

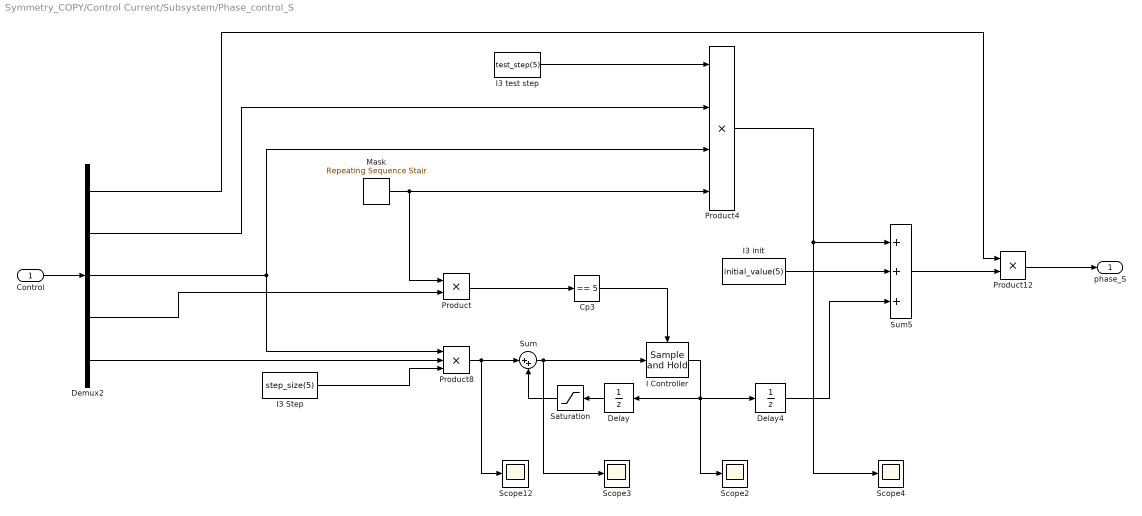
== system Symmetry_COPY/Control Current/Subsystem/Phase_control_S ==
  Control : Inport
  Cp3 : simulink/Logic and Bit Operations/Compare To Constant  relop===  const=5  OutDataTypeStr=uint8  ZeroCross=off
  Delay : UnitDelay  SampleTime=sample
  Delay4 : UnitDelay  SampleTime=sample
  Demux2 : Demux  Outputs=5
  I Controller : dspsigops/Sample and Hold  trig=Rising edge  initCond=0  latchinput=off
  I3 Step : Constant  Value=step_size(5)
  "I3 init " : Constant  Value=initial_value(5)
  I3 test step : Constant  Value=test_step(5)
  Mask : simulink/Sources/Repeating Sequence Stair  OutValues=[0 0 0 0 1 0].'  tsamp=0.02  OutMin=[]  OutMax=[]  OutDataTypeStr=float('double')  OutputDataTypeScalingMode=Specify via dialog  OutDataType=float('double')  ConRadixGroup=Best Precision: Vector-wise  OutScaling=2^-12
  Product : Product  RndMeth=Zero
  Product12 : Product  RndMeth=Zero
  Product4 : Product  Inputs=4  RndMeth=Zero
  Product8 : Product  Inputs=3  RndMeth=Zero
  Saturation : Saturate  UpperLimit=phase_feedback_saturation  LowerLimit=-phase_feedback_saturation
  Scope{2..4,12} (4 alike) : Scope
      Scope12 settings: YMin=-13  YMax=1  SaveName=ScopeData12
      Scope2 settings: SaveName=ScopeData4
      Scope3 settings: YMin=-13  YMax=1  SaveName=ScopeData5
  Sum : Sum  Inputs=|++
  Sum5 : Sum  Inputs=+++
  phase_S : Outport
  wires:
  Control/1 -> Demux2/1
  Product12/1 -> phase_S/1
  Product8/1 -> Sum/1, Scope12/1
  Delay/1 -> Saturation/1
  "I3 init "/1 -> Sum5/2
  Delay4/1 -> Sum5/3
  Demux2/5 -> Product8/2
  Demux2/4 -> Product/2
  Demux2/3 -> Product4/3, Product8/1
  Demux2/2 -> Product4/2
  Demux2/1 -> Product12/1
  I3 Step/1 -> Product8/3
  Cp3/1 -> I Controller/Trigger
  Mask/1 -> Product/1, Product4/4
  Sum5/1 -> Product12/2
  I3 test step/1 -> Product4/1
  I Controller/1 -> Delay4/1, Scope2/1, Delay/1
  Product4/1 -> Scope4/1, Sum5/1
  Product/1 -> Cp3/1
  Sum/1 -> I Controller/1, Scope3/1
  Saturation/1 -> Sum/2

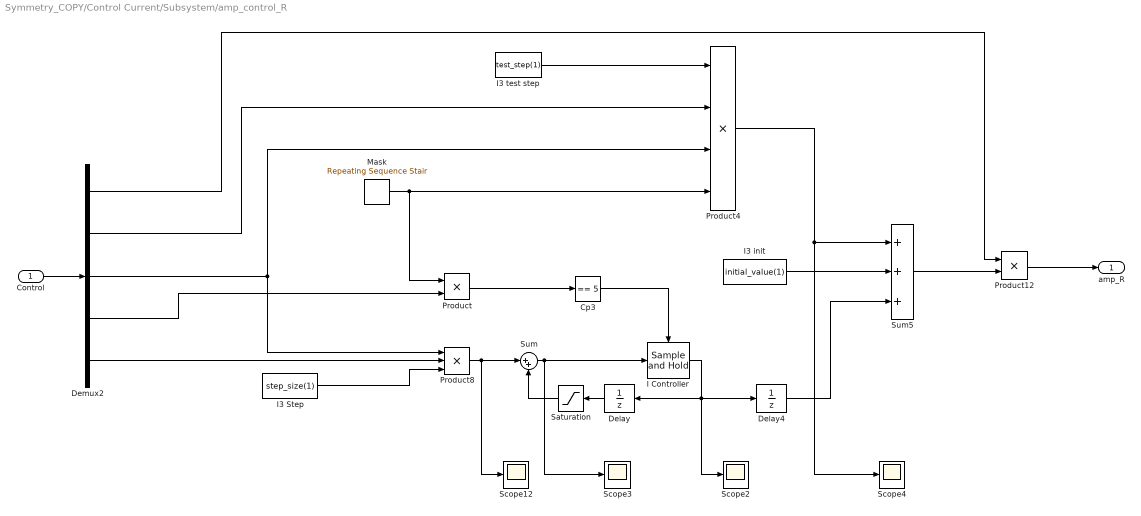
== system Symmetry_COPY/Control Current/Subsystem/amp_control_R ==
  Control : Inport
  Cp3 : simulink/Logic and Bit Operations/Compare To Constant  relop===  const=5  OutDataTypeStr=uint8  ZeroCross=off
  Delay : UnitDelay  SampleTime=sample
  Delay4 : UnitDelay  SampleTime=sample
  Demux2 : Demux  Outputs=5
  I Controller : dspsigops/Sample and Hold  trig=Rising edge  initCond=0  latchinput=off
  I3 Step : Constant  Value=step_size(1)
  "I3 init " : Constant  Value=initial_value(1)
  I3 test step : Constant  Value=test_step(1)
  Mask : simulink/Sources/Repeating Sequence Stair  OutValues=[1 0 0 0 0 0].'  tsamp=0.02  OutMin=[]  OutMax=[]  OutDataTypeStr=float('double')  OutputDataTypeScalingMode=Specify via dialog  OutDataType=float('double')  ConRadixGroup=Best Precision: Vector-wise  OutScaling=2^-12
  Product : Product  RndMeth=Zero
  Product12 : Product  RndMeth=Zero
  Product4 : Product  Inputs=4  RndMeth=Zero
  Product8 : Product  Inputs=3  RndMeth=Zero
  Saturation : Saturate  UpperLimit=amp_feedback_saturation  LowerLimit=-amp_feedback_saturation
  Scope{2..4,12} (4 alike) : Scope
      Scope12 settings: YMin=-13  YMax=1  SaveName=ScopeData12
      Scope2 settings: SaveName=ScopeData4
      Scope3 settings: YMin=-13  YMax=1  SaveName=ScopeData5
  Sum : Sum  Inputs=|++
  Sum5 : Sum  Inputs=+++
  amp_R : Outport
  wires:
  Control/1 -> Demux2/1
  Product12/1 -> amp_R/1
  Product8/1 -> Sum/1, Scope12/1
  Delay/1 -> Saturation/1
  "I3 init "/1 -> Sum5/2
  Delay4/1 -> Sum5/3
  Demux2/5 -> Product8/2
  Demux2/4 -> Product/2
  Demux2/3 -> Product4/3, Product8/1
  Demux2/2 -> Product4/2
  Demux2/1 -> Product12/1
  I3 Step/1 -> Product8/3
  Cp3/1 -> I Controller/Trigger
  Mask/1 -> Product/1, Product4/4
  Sum5/1 -> Product12/2
  I3 test step/1 -> Product4/1
  I Controller/1 -> Delay4/1, Scope2/1, Delay/1
  Product4/1 -> Scope4/1, Sum5/1
  Product/1 -> Cp3/1
  Sum/1 -> I Controller/1, Scope3/1
  Saturation/1 -> Sum/2

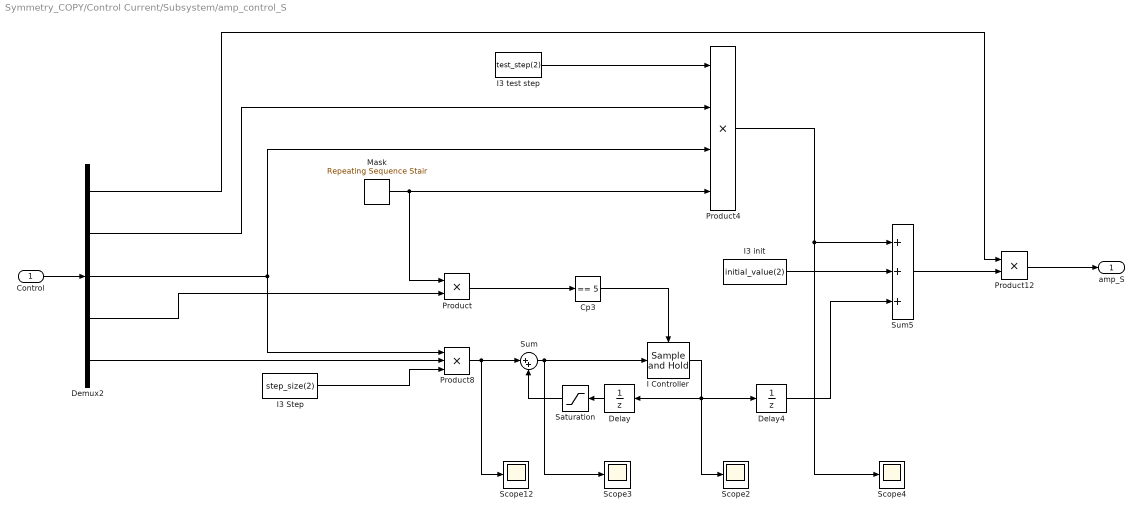
== system Symmetry_COPY/Control Current/Subsystem/amp_control_S ==
  Control : Inport
  Cp3 : simulink/Logic and Bit Operations/Compare To Constant  relop===  const=5  OutDataTypeStr=uint8  ZeroCross=off
  Delay : UnitDelay  SampleTime=sample
  Delay4 : UnitDelay  SampleTime=sample
  Demux2 : Demux  Outputs=5
  I Controller : dspsigops/Sample and Hold  trig=Rising edge  initCond=0  latchinput=off
  I3 Step : Constant  Value=step_size(2)
  "I3 init " : Constant  Value=initial_value(2)
  I3 test step : Constant  Value=test_step(2)
  Mask : simulink/Sources/Repeating Sequence Stair  OutValues=[0 1 0 0 0 0].'  tsamp=0.02  OutMin=[]  OutMax=[]  OutDataTypeStr=float('double')  OutputDataTypeScalingMode=Specify via dialog  OutDataType=float('double')  ConRadixGroup=Best Precision: Vector-wise  OutScaling=2^-12
  Product : Product  RndMeth=Zero
  Product12 : Product  RndMeth=Zero
  Product4 : Product  Inputs=4  RndMeth=Zero
  Product8 : Product  Inputs=3  RndMeth=Zero
  Saturation : Saturate  UpperLimit=amp_feedback_saturation  LowerLimit=-amp_feedback_saturation
  Scope{2..4,12} (4 alike) : Scope
      Scope12 settings: YMin=-13  YMax=1  SaveName=ScopeData12
      Scope2 settings: SaveName=ScopeData4
      Scope3 settings: YMin=-13  YMax=1  SaveName=ScopeData5
  Sum : Sum  Inputs=|++
  Sum5 : Sum  Inputs=+++
  amp_S : Outport
  wires:
  Saturation/1 -> Sum/2
  Sum/1 -> Scope3/1, I Controller/1
  Product/1 -> Cp3/1
  Product4/1 -> Sum5/1, Scope4/1
  I Controller/1 -> Delay/1, Scope2/1, Delay4/1
  I3 test step/1 -> Product4/1
  Sum5/1 -> Product12/2
  Mask/1 -> Product4/4, Product/1
  Cp3/1 -> I Controller/Trigger
  I3 Step/1 -> Product8/3
  Demux2/1 -> Product12/1
  Demux2/2 -> Product4/2
  Demux2/3 -> Product8/1, Product4/3
  Demux2/4 -> Product/2
  Demux2/5 -> Product8/2
  Delay4/1 -> Sum5/3
  "I3 init "/1 -> Sum5/2
  Delay/1 -> Saturation/1
  Product8/1 -> Scope12/1, Sum/1
  Product12/1 -> amp_S/1
  Control/1 -> Demux2/1

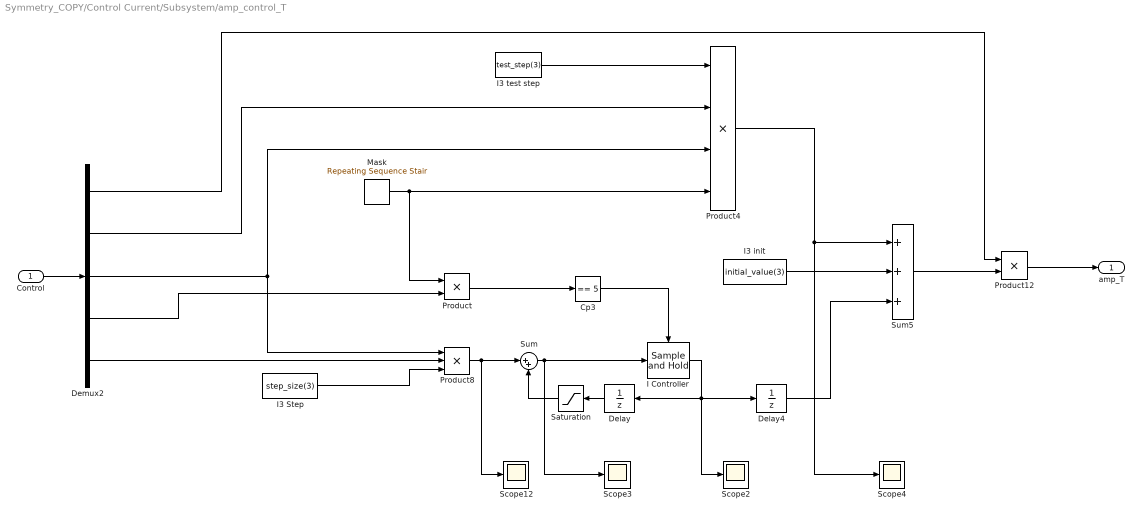
== system Symmetry_COPY/Control Current/Subsystem/amp_control_T ==
  Control : Inport
  Cp3 : simulink/Logic and Bit Operations/Compare To Constant  relop===  const=5  OutDataTypeStr=uint8  ZeroCross=off
  Delay : UnitDelay  SampleTime=sample
  Delay4 : UnitDelay  SampleTime=sample
  Demux2 : Demux  Outputs=5
  I Controller : dspsigops/Sample and Hold  trig=Rising edge  initCond=0  latchinput=off
  I3 Step : Constant  Value=step_size(3)
  "I3 init " : Constant  Value=initial_value(3)
  I3 test step : Constant  Value=test_step(3)
  Mask : simulink/Sources/Repeating Sequence Stair  OutValues=[0 0 1 0 0 0].'  tsamp=0.02  OutMin=[]  OutMax=[]  OutDataTypeStr=float('double')  OutputDataTypeScalingMode=Specify via dialog  OutDataType=float('double')  ConRadixGroup=Best Precision: Vector-wise  OutScaling=2^-12
  Product : Product  RndMeth=Zero
  Product12 : Product  RndMeth=Zero
  Product4 : Product  Inputs=4  RndMeth=Zero
  Product8 : Product  Inputs=3  RndMeth=Zero
  Saturation : Saturate  UpperLimit=amp_feedback_saturation  LowerLimit=-amp_feedback_saturation
  Scope{2..4,12} (4 alike) : Scope
      Scope12 settings: YMin=-13  YMax=1  SaveName=ScopeData12
      Scope2 settings: SaveName=ScopeData4
      Scope3 settings: YMin=-13  YMax=1  SaveName=ScopeData5
  Sum : Sum  Inputs=|++
  Sum5 : Sum  Inputs=+++
  amp_T : Outport
  wires:
  Control/1 -> Demux2/1
  Product12/1 -> amp_T/1
  Product8/1 -> Sum/1, Scope12/1
  Delay/1 -> Saturation/1
  "I3 init "/1 -> Sum5/2
  Delay4/1 -> Sum5/3
  Demux2/5 -> Product8/2
  Demux2/4 -> Product/2
  Demux2/3 -> Product4/3, Product8/1
  Demux2/2 -> Product4/2
  Demux2/1 -> Product12/1
  I3 Step/1 -> Product8/3
  Cp3/1 -> I Controller/Trigger
  Mask/1 -> Product/1, Product4/4
  Sum5/1 -> Product12/2
  I3 test step/1 -> Product4/1
  I Controller/1 -> Delay4/1, Scope2/1, Delay/1
  Product4/1 -> Scope4/1, Sum5/1
  Product/1 -> Cp3/1
  Sum/1 -> I Controller/1, Scope3/1
  Saturation/1 -> Sum/2

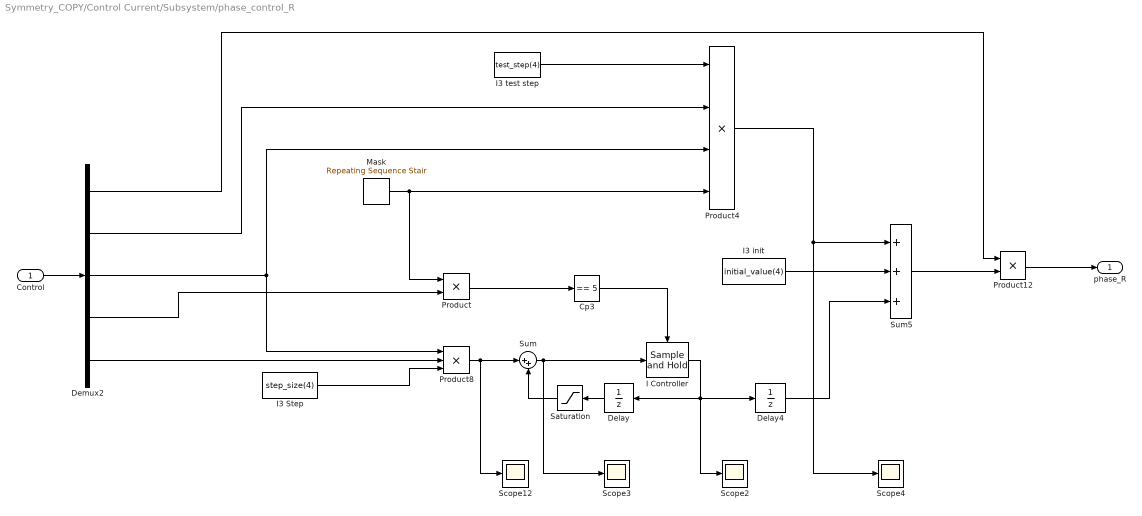
== system Symmetry_COPY/Control Current/Subsystem/phase_control_R ==
  Control : Inport
  Cp3 : simulink/Logic and Bit Operations/Compare To Constant  relop===  const=5  OutDataTypeStr=uint8  ZeroCross=off
  Delay : UnitDelay  SampleTime=sample
  Delay4 : UnitDelay  SampleTime=sample
  Demux2 : Demux  Outputs=5
  I Controller : dspsigops/Sample and Hold  trig=Rising edge  initCond=0  latchinput=off
  I3 Step : Constant  Value=step_size(4)
  "I3 init " : Constant  Value=initial_value(4)
  I3 test step : Constant  Value=test_step(4)
  Mask : simulink/Sources/Repeating Sequence Stair  OutValues=[0 0 0 1 0 0].'  tsamp=0.02  OutMin=[]  OutMax=[]  OutDataTypeStr=float('double')  OutputDataTypeScalingMode=Specify via dialog  OutDataType=float('double')  ConRadixGroup=Best Precision: Vector-wise  OutScaling=2^-12
  Product : Product  RndMeth=Zero
  Product12 : Product  RndMeth=Zero
  Product4 : Product  Inputs=4  RndMeth=Zero
  Product8 : Product  Inputs=3  RndMeth=Zero
  Saturation : Saturate  UpperLimit=phase_feedback_saturation  LowerLimit=-phase_feedback_saturation
  Scope{2..4,12} (4 alike) : Scope
      Scope12 settings: YMin=-13  YMax=1  SaveName=ScopeData12
      Scope2 settings: SaveName=ScopeData4
      Scope3 settings: YMin=-13  YMax=1  SaveName=ScopeData5
  Sum : Sum  Inputs=|++
  Sum5 : Sum  Inputs=+++
  phase_R : Outport
  wires:
  Saturation/1 -> Sum/2
  Sum/1 -> Scope3/1, I Controller/1
  Product/1 -> Cp3/1
  Product4/1 -> Sum5/1, Scope4/1
  I Controller/1 -> Delay/1, Scope2/1, Delay4/1
  I3 test step/1 -> Product4/1
  Sum5/1 -> Product12/2
  Mask/1 -> Product4/4, Product/1
  Cp3/1 -> I Controller/Trigger
  I3 Step/1 -> Product8/3
  Demux2/1 -> Product12/1
  Demux2/2 -> Product4/2
  Demux2/3 -> Product8/1, Product4/3
  Demux2/4 -> Product/2
  Demux2/5 -> Product8/2
  Delay4/1 -> Sum5/3
  "I3 init "/1 -> Sum5/2
  Delay/1 -> Saturation/1
  Product8/1 -> Scope12/1, Sum/1
  Product12/1 -> phase_R/1
  Control/1 -> Demux2/1

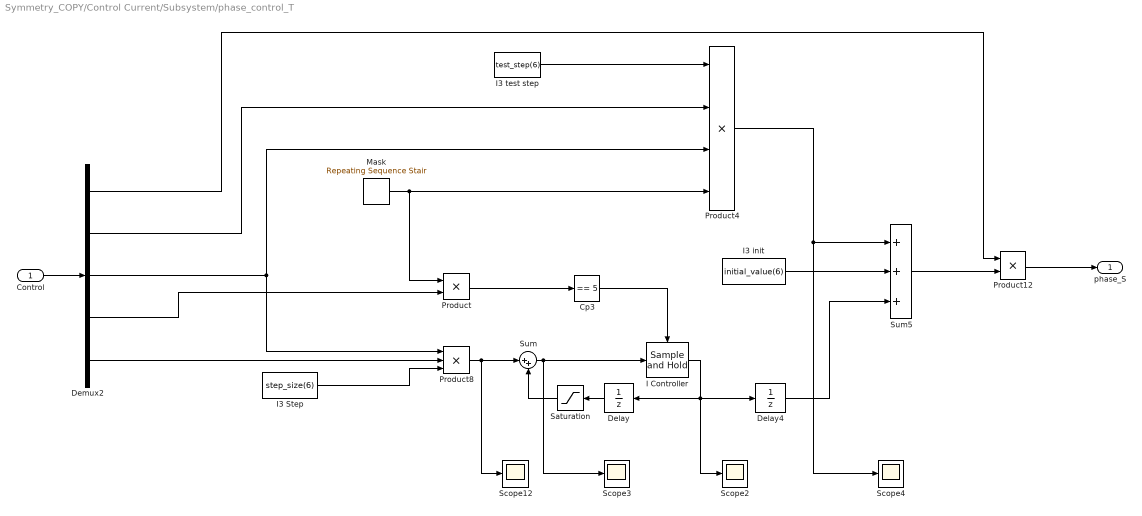
== system Symmetry_COPY/Control Current/Subsystem/phase_control_T ==
  Control : Inport
  Cp3 : simulink/Logic and Bit Operations/Compare To Constant  relop===  const=5  OutDataTypeStr=uint8  ZeroCross=off
  Delay : UnitDelay  SampleTime=sample
  Delay4 : UnitDelay  SampleTime=sample
  Demux2 : Demux  Outputs=5
  I Controller : dspsigops/Sample and Hold  trig=Rising edge  initCond=0  latchinput=off
  I3 Step : Constant  Value=step_size(6)
  "I3 init " : Constant  Value=initial_value(6)
  I3 test step : Constant  Value=test_step(6)
  Mask : simulink/Sources/Repeating Sequence Stair  OutValues=[0 0 0 0 0 1].'  tsamp=0.02  OutMin=[]  OutMax=[]  OutDataTypeStr=float('double')  OutputDataTypeScalingMode=Specify via dialog  OutDataType=float('double')  ConRadixGroup=Best Precision: Vector-wise  OutScaling=2^-12
  Product : Product  RndMeth=Zero
  Product12 : Product  RndMeth=Zero
  Product4 : Product  Inputs=4  RndMeth=Zero
  Product8 : Product  Inputs=3  RndMeth=Zero
  Saturation : Saturate  UpperLimit=phase_feedback_saturation  LowerLimit=-phase_feedback_saturation
  Scope{2..4,12} (4 alike) : Scope
      Scope12 settings: YMin=-13  YMax=1  SaveName=ScopeData12
      Scope2 settings: SaveName=ScopeData4
      Scope3 settings: YMin=-13  YMax=1  SaveName=ScopeData5
  Sum : Sum  Inputs=|++
  Sum5 : Sum  Inputs=+++
  phase_S : Outport
  wires:
  Saturation/1 -> Sum/2
  Sum/1 -> Scope3/1, I Controller/1
  Product/1 -> Cp3/1
  Product4/1 -> Sum5/1, Scope4/1
  I Controller/1 -> Delay/1, Scope2/1, Delay4/1
  I3 test step/1 -> Product4/1
  Sum5/1 -> Product12/2
  Mask/1 -> Product4/4, Product/1
  Cp3/1 -> I Controller/Trigger
  I3 Step/1 -> Product8/3
  Demux2/1 -> Product12/1
  Demux2/2 -> Product4/2
  Demux2/3 -> Product8/1, Product4/3
  Demux2/4 -> Product/2
  Demux2/5 -> Product8/2
  Delay4/1 -> Sum5/3
  "I3 init "/1 -> Sum5/2
  Delay/1 -> Saturation/1
  Product8/1 -> Scope12/1, Sum/1
  Product12/1 -> phase_S/1
  Control/1 -> Demux2/1

== system Symmetry_COPY/Load System/Loads/Capacitive_Loads_RST ==
  Breaker1 : powerlib/Elements/Breaker  BreakerResistance=0.01  InitialState=0  SnubberResistance=1e7  SnubberCapacitance=inf  SwitchingTimes="[ 1/60  5/60 ]"  External=on  Measurements=None  MoreParameters=off  NoBreakLoop=off
  Breaker4 : powerlib/Elements/Breaker  BreakerResistance=0.01  InitialState=0  SnubberResistance=1e7  SnubberCapacitance=inf  SwitchingTimes="[ 1/60  5/60 ]"  External=on  Measurements=None  MoreParameters=off  NoBreakLoop=off
  Breaker6 : powerlib/Elements/Breaker  BreakerResistance=0.01  InitialState=0  SnubberResistance=1e7  SnubberCapacitance=inf  SwitchingTimes="[ 1/60  5/60 ]"  External=on  Measurements=None  MoreParameters=off  NoBreakLoop=off
  Capacitive_Load_R : Subsystem
  Capacitive_Load_S : Subsystem
  Capacitive_Load_T : Subsystem
  NL Loads On grid : Constant  Value=Switch_Load_RC(1)
  NL Loads On grid1 : Constant  Value=Switch_Load_RC(2)
  NL Loads On grid2 : Constant  Value=Switch_Load_RC(3)
  R : PMIOPort  Port=1  Side=Right
  S : PMIOPort  Port=2  Side=Right
  T : PMIOPort  Port=3  Side=Right
  N : PMIOPort  Port=4  Side=Left
  wires:
  NL Loads On grid/1 -> Breaker4/1
  NL Loads On grid1/1 -> Breaker1/1
  NL Loads On grid2/1 -> Breaker6/1
  connections:
  R/RConn1 -- Breaker4/LConn1
  S/RConn1 -- Breaker1/LConn1
  T/RConn1 -- Breaker6/LConn1
  Capacitive_Load_R/LConn1 -- Breaker4/RConn1
  Capacitive_Load_S/LConn1 -- Breaker1/RConn1
  Capacitive_Load_T/LConn1 -- Breaker6/RConn1
  Capacitive_Load_R/LConn2 -- Capacitive_Load_S/LConn2 -- Capacitive_Load_T/LConn2 -- N/RConn1
